simulink model "Final_Model_Building_2_AirflowAdded_BufferMode"  (R2022a)
settings: Solver=FixedStepAuto  StartTime=0.0  StopTime=24*3600  FixedStep=5  RelTol=1e-3
values from neighbouring files (symbols this model uses):
  Aux_Threshold = 52    [Setup_Code_EWASP_VC.m]
  buildingAge = 2005    [Setup_Code_EWASP_VC.m]
  ceilingHeight = 2.4    [Setup_Code_EWASP_VC.m]
  conductiveHconnectMatrix = [ ... (first row only)    [Setup_Code_EWASP_VC.m]
  cRoofGreen = 100000    [Setup_Code_EWASP_VC.m]
  Defrost_After_Time = 30    [Setup_Code_EWASP_VC.m]
  DHWDemandProfile = occFreegainHotwaterElecTestPassiveOcc3(:,3)    [Setup_Code_EWASP_VC.m]
  Elec_Max = Elec_Max*(30/24.2)    [Setup_Code_EWASP_VC.m]
  Elec_Mid = Elec_Mid*(30/24.2)    [Setup_Code_EWASP_VC.m]
  Elec_Min = Elec_Min*(30/24.2)    [Setup_Code_EWASP_VC.m]
  ElecDemandProfile = occFreegainHotwaterElecTestPassiveOcc3(:,4)    [Setup_Code_EWASP_VC.m]
  ElecFixed = [Elec_Max(6,2) Elec_Max(6,4) Elec_Max(6,6) Elec_Max(6,7) ... (first row only)    [Setup_Code_EWASP_VC.m]
  floorOrCeilingArea = floorOrCeilingArea*1.15    [Setup_Code_EWASP_VC.m]
  freegain = occFreegainHotwaterElecTestPassiveOcc3(:,2)-max(occupancy)*25    [Setup_Code_EWASP_VC.m]
  furnitureModelOn = 1    [Setup_Code_EWASP_VC.m]
  Heat_Max = Heat_Max*(30/24.2)    [Setup_Code_EWASP_VC.m]
  Heat_Mid = Heat_Mid*(30/24.2)    [Setup_Code_EWASP_VC.m]
  Heat_Min = Heat_Min*(30/24.2)    [Setup_Code_EWASP_VC.m]
  HeatFixed = [Heat_Max(6,2) Heat_Max(6,4) Heat_Max(6,6) Heat_Max(6,7) ... (first row only)    [Setup_Code_EWASP_VC.m]
  HeatingOnProfile = repmat(HeatingOnProfile,365,1)    [Setup_Code_EWASP_VC.m]
  HEX_ReturnLowerLimit = 52.5    [Setup_Code_EWASP_VC.m]
  HEX_ReturnUpperLimit = 55    [Setup_Code_EWASP_VC.m]
  LeakMultiplier = 1+(2*(rand()-0.5)/10)    [Setup_Code_EWASP_VC.m]
  maxOcc = max(occupancyProfile)    [Setup_Code_EWASP_VC.m]
  NESW_wallArea = max(NESW_Lengths*ceilingHeight-NESW_Windows,0)    [Setup_Code_EWASP_VC.m]
  NESW_Windows = [ ... (first row only)    [Setup_Code_EWASP_VC.m]
  numRooms = roomCount    [Setup_Code_EWASP_VC.m]
  occupancy = occupancyProfile    [Setup_Code_EWASP_VC.m]
  offsetDays = 0    [Setup_Code_EWASP_VC.m]
  overChargeSeries = repmat(overChargeSeries,365,1)    [Setup_Code_EWASP_VC.m]
  pumpChoice = pumpChoices(MinIndex,1)    [Setup_Code_EWASP_VC.m]
  pumpRamp = 180    [Setup_Code_EWASP_VC.m]
  RoofIrradiance = Flat_NS_EW_RoofIrradiance(:,1)    [Setup_Code_EWASP_VC.m]
  roofStartTemp = ones(11,1)*20    [Setup_Code_EWASP_VC.m]
  rooftype = 0    [Setup_Code_EWASP_VC.m]
  RoomDataMatrix = [zeros(1,12);ones(1,12)*wallDensity;zeros(1,12);ones(1,12)*wallU;ones(1,12)*windowU;ones(1,12)*floorU;ones(1,12)*ceilingU;zeros(1,12);windowArea, 0;floorOrCeilingArea;zeros(1,12);floorOrCeilingArea*ceilingHeight]    [Setup_Code_EWASP_VC.m]
  roomVol = roomVol*1.15    [Setup_Code_EWASP_VC.m]
  slabStartTemp = (GroundTempTimeSeries(offsetDays*1440+1,1)+thermostatSetting)/2    [Setup_Code_EWASP_VC.m]
  SlackRequest = zeros(1440,1)    [Setup_Code_EWASP_VC.m]
  SolarThermalExists = 0    [Setup_Code_EWASP_VC.m]
  SourceFixed = HeatFixed-ElecFixed    [Setup_Code_EWASP_VC.m]
  StateSeries = StateSeriesGenerator(22,7,1)    [Setup_Code_EWASP_VC.m]
  Tank_Lower_Temp = 49.5    [Setup_Code_EWASP_VC.m]
  Tank_Upper_Temp = 52    [Setup_Code_EWASP_VC.m]
  Tank_Volume_m3 = 0.15    [Setup_Code_EWASP_VC.m]
  TankHeatHour = randi([1 5])-1    [Setup_Code_EWASP_VC.m]
  upDown = [0;0;0;0;1;1;1;1;1;1;1]    [Setup_Code_EWASP_VC.m]
  wallStartTempExt = thermostatSetting*(0.266+0.00215*outdoorStartTemp+0.018*wallU+0.00113*outdoorStartTemp*wallU+0.0068*wallU^2)    [Setup_Code_EWASP_VC.m]
undefined symbols (not defined in the file or in its folder): a, ceilingU, condUDMatrix, convUDMatrix, deltaPEXPANDED_E, deltaPEXPANDED_E2, deltaPEXPANDED_N, deltaPEXPANDED_N2, deltaPEXPANDED_S, deltaPEXPANDED_S2, deltaPEXPANDED_W, deltaPEXPANDED_W2, DesiredDHWTemp, DesiredFlowTempVsInOutDeltaTemp, DiffuseHorizontal, DiscIntNeverNeededParam, DNI, dwnAndConcrete, ExtractRates, GroundTempTimeSeries, HCM, HCM2, HCM_closed, HCM_closed2, intermediateU, IsTop, massFlowMatrix, mechEfficiency, neighbourMatrix, numericalRoomUse, RadiatorMatrix, room2roomflowmatrix_E, room2roomflowmatrix_E2, room2roomflowmatrix_N, room2roomflowmatrix_N2, room2roomflowmatrix_S, room2roomflowmatrix_S2, room2roomflowmatrix_W, room2roomflowmatrix_W2, StateAirInEXPANDED_E, StateAirInEXPANDED_E2, StateAirInEXPANDED_N, StateAirInEXPANDED_N2, StateAirInEXPANDED_S, StateAirInEXPANDED_S2, StateAirInEXPANDED_W, StateAirInEXPANDED_W2, StateAirOutEXPANDED_E, StateAirOutEXPANDED_E2, StateAirOutEXPANDED_N, StateAirOutEXPANDED_N2, StateAirOutEXPANDED_S, StateAirOutEXPANDED_S2, StateAirOutEXPANDED_W, StateAirOutEXPANDED_W2, tankExists, TemperatureSeries, ThermostatBand, ThermostatSetting, Tin1 ... (+10)
libraries: simulink x6, dspsigops x4, dspmtrx3 x4, powerlib_meascontrol x3, carnot x3, dspstat3 x2
(part 3 of 29)

== system Final_Model_Building_2_AirflowAdded_BufferMode/Subsystem4 ==
  note: roof masses (45kg/m^2) and heat capacities calculated
      | using https://www.steelbeamcalculator.co.uk/standardloads
  In1 : Inport
  In2 : Inport  Port=2
  In3 : Inport  Port=3
  Ceil node tmperatures : DiscreteIntegrator  InitialConditionSource=external  InitialCondition=20  SampleTime=-1  ICPrevOutput=DiscIntNeverNeededParam  ICPrevScaledInput=DiscIntNeverNeededParam
  Display1 : Display
  Divide : Product  Inputs=*/
  Divide1 : Product  Inputs=*/
  Heat to ceilingNodes : Product  Inputs=4
  Heat to roofspace airnode : Sum  Inputs=+
  Heatloss roof to environment : Subsystem
  MATLAB Function1 : MATLAB Function  TreatAsAtomicUnit=on
  MATLAB Function2 : MATLAB Function  TreatAsAtomicUnit=on
  MATLAB Function3 : MATLAB Function  TreatAsAtomicUnit=on
  MATLAB Function4 : MATLAB Function  TreatAsAtomicUnit=on
  Product1 : Product  Inputs=3
  "Roof Temp " : DiscreteIntegrator  InitialConditionSource=external  InitialCondition=20  SampleTime=-1  ICPrevOutput=DiscIntNeverNeededParam  ICPrevScaledInput=DiscIntNeverNeededParam
  "RoofspaceTemp " : DiscreteIntegrator  InitialConditionSource=external  InitialCondition=20  SampleTime=-1  ICPrevOutput=DiscIntNeverNeededParam  ICPrevScaledInput=DiscIntNeverNeededParam
  Subtract : Sum  Inputs=+-
  Subtract1 : Sum
  Subtract2 : Sum  Inputs=+-
  Subtract3 : Sum  Inputs=+-
  Subtract4 : Sum  Inputs=2
  Subtract5 : Sum  Inputs=-+
  Total roofstructure heat capacity : Product
  Unary Minus : UnaryMinus
  air density per m3 : Constant  Value=1.225
  air heat capacity per kg : Constant  Value=1000
  ceiling heatchange due to loss to roofspace : UnaryMinus
  ceilnode heat capacities(predominantly plaster mass) : Constant  Value=10*1090*(IsTop(1:1:11)').*floorOrCeilingArea(1:1:11)'
  ceilnode heat capacities(predominantly plaster mass)1 : Constant  Value=10*1090*(IsTop(1,1:11)').*floorOrCeilingArea(1,1:11)'
  convective transfer to ceiling node : Constant  Value=2
  deltaTCeilingNodes : Product  Inputs=*/
  deltaTCeilingNodes1 : Product  Inputs=*/
  estimate of pitched roofspace air volume: 0.5 * floorArea of loft * height at peak : Constant  Value=0.5*sum(floorOrCeilingArea(1,1:11)'.*IsTop(1,1:11)')*(0.5*(sum(floorOrCeilingArea(1,1:11)'.*IsTop(1,1:11)')).^0.5)
  heat loss ceiing to roofspace : Product
  heat loss roofspace to roof : Product
  initial ceilnode temps : Constant  Value=20*ones(11,1)
  initial ceilnode temps1 : Constant  Value=10
  initial ceilnode temps2 : Constant  Value=10
  mass of roof per m^2*predictedroofarea : Constant  Value=45*sum(floorOrCeilingArea(1,1:11)'.*IsTop(1,1:11)')*1.414
  roofspace heatchange due to loss to roof : UnaryMinus
  room is on the top floor : Constant  Value=IsTop(1,1:11)'
  room is on the top floor1 : Constant  Value=floorOrCeilingArea(1,1:11)'
  slate heat capacity per kg1 : Constant  Value=760
  w/k loss from ceiling to roofspace : Constant  Value=(ceilingU*2)*(floorOrCeilingArea(1,1:11)').*(IsTop(1,1:11)')
  w/k loss from roofspace to roof : Constant  Value=(ceilingU*2)*sum(floorOrCeilingArea(1,1:11)'.*IsTop(1,1:11)')*1.414
  Out1 : Outport  VectorParamsAs1DForOutWhenUnconnected=off
  wires:
  In2/1 -> [windSpeed]
  In1/1 -> Subtract/1
  Subtract5/1 -> Divide1/1
  w/k loss from roofspace to roof/1 -> heat loss roofspace to roof/2
  Subtract/1 -> Heat to ceilingNodes/1
  Product1/1 -> Divide/2
  estimate of pitched roofspace air volume: 0.5 * floorArea of loft * height at peak/1 -> Product1/2
  air heat capacity per kg/1 -> Product1/3
  room is on the top floor/1 -> Heat to ceilingNodes/2
  heat loss roofspace to roof/1 -> roofspace heatchange due to loss to roof/1, Subtract5/2
  MATLAB Function3/1(y) -> Subtract1/2
  convective transfer to ceiling node/1 -> Heat to ceilingNodes/4
  air density per m3/1 -> Product1/1
  initial ceilnode temps1/1 -> "RoofspaceTemp "/2
  Heatloss roof to environment/1(Out1) -> Subtract5/1
  Heat to roofspace airnode/1 -> Display1/1, Subtract4/1
  Total roofstructure heat capacity/1 -> Divide1/2
  slate heat capacity per kg1/1 -> Total roofstructure heat capacity/1
  deltaTCeilingNodes1/1 -> MATLAB Function3/1(u)
  ceilnode heat capacities(predominantly plaster mass)1/1 -> deltaTCeilingNodes1/2
  MATLAB Function4/1(y) -> "Roof Temp "/1
  w/k loss from ceiling to roofspace/1 -> heat loss ceiing to roofspace/2
  deltaTCeilingNodes/1 -> MATLAB Function1/1(u)
  Subtract4/1 -> Divide/1
  Subtract3/1 -> heat loss roofspace to roof/1
  MATLAB Function2/1(y) -> "RoofspaceTemp "/1
  room is on the top floor1/1 -> Heat to ceilingNodes/3
  Ceil node tmperatures/1 -> Subtract2/1, Subtract/2
  mass of roof per m^2*predictedroofarea/1 -> Total roofstructure heat capacity/2
  ceilnode heat capacities(predominantly plaster mass)/1 -> deltaTCeilingNodes/2
  ceiling heatchange due to loss to roofspace/1 -> deltaTCeilingNodes1/1
  [windSpeed] -> Heatloss roof to environment/1(In1)
  initial ceilnode temps2/1 -> "Roof Temp "/2
  Heat to ceilingNodes/1 -> Unary Minus/1, deltaTCeilingNodes/1
  MATLAB Function1/1(y) -> Subtract1/1
  In3/1 -> [outdoorTemp]
  roofspace heatchange due to loss to roof/1 -> Subtract4/2
  Subtract2/1 -> heat loss ceiing to roofspace/1
  Divide1/1 -> MATLAB Function4/1(u)
  Divide/1 -> MATLAB Function2/1(u)
  "RoofspaceTemp "/1 -> Subtract3/1, Subtract2/2
  [outdoorTemp] -> Heatloss roof to environment/2(In2)
  Subtract1/1 -> Ceil node tmperatures/1
  initial ceilnode temps/1 -> Ceil node tmperatures/2
  heat loss ceiing to roofspace/1 -> ceiling heatchange due to loss to roofspace/1, Heat to roofspace airnode/1
  "Roof Temp "/1 -> Subtract3/2, Heatloss roof to environment/3(In3)
  Unary Minus/1 -> Out1/1

== system Final_Model_Building_2_AirflowAdded_BufferMode/Subsystem_Room1 ==
  DNI1 : Constant  Value=50
  Diffuse Irradiance1 : Constant  Value=50
  Ground : Ground
  Incidence Angle1 : Constant  Value=60
  Integrator : Integrator  InitialConditionSource=external  InitialCondition=Tin1
  Lounge/Dining : Subsystem
      mask Display:
      | port_label('input', 1, 'THB in')
      | port_label('input', 2, 'Mdot_Rad_Full_open')
      | port_label('input', 3, 'T In')
      | port_label('input', 4, 'T Out')
      | port_label('input', 5, 'T up (conv)')
      | port_label('input', 6, 'T Down (conv)')
      | port_label('input', 7, 'T Bel (cond)')
      | port_label('input', 8, 'T Abv (cond)')
      | port_label('input', 9, 'T N1')
      | port_label('input', 10, 'T N2')
      | port_label('input', 11, 'T N3')
      | port_label('input', 12, 'T N4')
      | port_label('input', 13, 'T N5')
      | port_label('input', 14, 'T Wall')
      | port_label('input', 15, 'Ang')
      | port_label('input', 16, 'Tilt')
      | port_label('input', 17, 'DNI')
      | port_label('input', 18, 'DiffI')
      | 
      | port_label('output', 1, 'THB Out')
      | port_label('output', 2, 'DeltaT Wall')
      | port_label('output', 3, 'DeltaT Room')
      | port_label('output', 5, 'Mdot_Actual')
  Panel TIlt1 : Constant  Value=90
  Subsystem11 : Subsystem
      mask Display:
      | disp('Vertical \n Conductive \n Signalling \n Block')
      | port_label('input', 1, 'Bel1')
      | port_label('input', 2, 'Bel2')
      | port_label('input', 3, 'Abv1')
      | port_label('input', 4, 'Abv2')
      | 
      | port_label('output', 1, 'T Bel')
      | port_label('output', 2, 'T Abv')
  Subsystem3 : Subsystem
      mask Display:
      | disp('Horizontal \n Neighbour \n Signalling \n Block')
      | port_label('input', 1, 'Nbr1')
      | port_label('input', 2, 'Nbr2')
      | port_label('input', 3, 'Nbr3')
      | port_label('input', 4, 'Nbr4')
      | port_label('input', 5, 'Nbr5')
      | port_label('output', 1, 'TN1')
      | port_label('output', 2, 'TN2')
      | port_label('output', 3, 'TN3')
      | port_label('output', 4, 'TN4')
      | port_label('output', 5, 'TN5')
  Terminator14 : Terminator
  Terminator2 : Terminator
  Tinitial1 : Constant  Value=21
  Twall11 : Constant  Value=neighbourMatrix(1,1)
  Twall12 : Constant  Value=neighbourMatrix(2,1)
  Twall13 : Constant  Value=neighbourMatrix(3,1)
  Twall14 : Constant  Value=neighbourMatrix(4,1)
  Twall15 : Constant  Value=neighbourMatrix(5,1)
  Twall33 : Constant  Value=condUDMatrix(1,1)
  Twall34 : Constant  Value=condUDMatrix(2,1)
  Twall35 : Constant  Value=condUDMatrix(3,1)
  Twall36 : Constant  Value=condUDMatrix(4,1)
  tag scope: DeltaT_1=global, Mdot_Actual_1=global, T_1=global, T_return_R1=global
  wires:
  [T_Out] -> Lounge/Dining/4(In3)
  Subsystem11/1(Out1) -> Lounge/Dining/7(In6)
  [T_1] -> Lounge/Dining/3(In2)
  Incidence Angle1/1 -> Lounge/Dining/15(In14)
  DNI1/1 -> Lounge/Dining/17(In16)
  Twall34/1 -> Subsystem11/2(In2)
  Subsystem3/5(Out5) -> Lounge/Dining/13(In12)
  Twall36/1 -> Subsystem11/4(In4)
  Twall33/1 -> Subsystem11/1(In1)
  Tinitial1/1 -> Integrator/2
  [DeltaT_1] -> Integrator/1
  [T_1] -> Lounge/Dining/5(In4), Lounge/Dining/6(In5)
  Twall11/1 -> Subsystem3/1(In1)
  Lounge/Dining/5(Out5) -> [Mdot_Actual_1]
  Subsystem3/1(Out1) -> Lounge/Dining/9(In8)
  Lounge/Dining/3(Out3) -> [DeltaT_1]
  Lounge/Dining/1(Out1) -> [T_return_R1]
  Lounge/Dining/4(Out4) -> Terminator2/1
  Diffuse Irradiance1/1 -> Lounge/Dining/18(In17)
  Lounge/Dining/2(Out2) -> Terminator14/1
  [THB_In] -> Lounge/Dining/1(In1)
  [MassFlow_Full_Open_1] -> Lounge/Dining/2(In18)
  Subsystem3/4(Out4) -> Lounge/Dining/12(In11)
  Twall13/1 -> Subsystem3/3(In3)
  Subsystem3/3(Out3) -> Lounge/Dining/11(In10)
  Twall15/1 -> Subsystem3/5(In5)
  Subsystem11/2(Out2) -> Lounge/Dining/8(In7)
  Ground/1 -> Lounge/Dining/14(In13)
  Twall14/1 -> Subsystem3/4(In4)
  Panel TIlt1/1 -> Lounge/Dining/16(In15)
  Integrator/1 -> [T_1]
  Twall12/1 -> Subsystem3/2(In2)
  Subsystem3/2(Out2) -> Lounge/Dining/10(In9)
  Twall35/1 -> Subsystem11/3(In3)

== system Final_Model_Building_2_AirflowAdded_BufferMode/Subsystem_Room10 ==
  DNI15 : Constant  Value=0
  Diffuse Irradiance10 : Constant  Value=0
  En suite : Subsystem
      mask Display:
      | port_label('input', 1, 'THB in')
      | port_label('input', 2, 'T In')
      | port_label('input', 3, 'T Out')
      | port_label('input', 4, 'T up (conv)')
      | port_label('input', 5, 'T Down (conv)')
      | port_label('input', 6, 'T Bel (cond)')
      | port_label('input', 7, 'T Abv (cond)')
      | port_label('input', 8, 'T N1')
      | port_label('input', 9, 'T N2')
      | port_label('input', 10, 'T N3')
      | port_label('input', 11, 'T N4')
      | port_label('input', 12, 'T N5')
      | port_label('input', 13, 'T Wall')
      | port_label('input', 14, 'Ang')
      | port_label('input', 15, 'Tilt')
      | port_label('input', 16, 'DNI')
      | port_label('input', 17, 'DiffI')
      | 
      | port_label('output', 1, 'THB Out')
      | port_label('output', 2, 'DeltaT Wall')
      | port_label('output', 3, 'DeltaT Room')
      | 
      | port_label('input', 18, 'm_dot_Fully_open')
      | port_label('output', 5, 'm_dot_Actual')
  Ground6 : Ground
  Incidence Angle10 : Constant  Value=60
  Integrator20 : Integrator  InitialConditionSource=external  InitialCondition=Tin1
  Panel TIlt10 : Constant  Value=90
  Scope34 : Scope
  Subsystem12 : Subsystem
      mask Display:
      | disp('Horizontal \n Neighbour \n Signalling \n Block')
      | port_label('input', 1, 'Nbr1')
      | port_label('input', 2, 'Nbr2')
      | port_label('input', 3, 'Nbr3')
      | port_label('input', 4, 'Nbr4')
      | port_label('input', 5, 'Nbr5')
      | port_label('output', 1, 'TN1')
      | port_label('output', 2, 'TN2')
      | port_label('output', 3, 'TN3')
      | port_label('output', 4, 'TN4')
      | port_label('output', 5, 'TN5')
  Subsystem23 : Subsystem
      mask Display:
      | disp('Vertical \n Convective \n Signalling \n Block')
      | port_label('input', 1, 'Nbr1')
      | port_label('input', 2, 'Nbr2')
      | 
      | port_label('output', 1, 'Tup')
      | port_label('output', 2, 'Tdwn')
  Subsystem28 : Subsystem
      mask Display:
      | disp('Vertical \n Conductive \n Signalling \n Block')
      | port_label('input', 1, 'Bel1')
      | port_label('input', 2, 'Bel2')
      | port_label('input', 3, 'Abv1')
      | port_label('input', 4, 'Abv2')
      | 
      | port_label('output', 1, 'T Bel')
      | port_label('output', 2, 'T Abv')
  Terminator7 : Terminator
  Tinitial14 : Constant  Value=20
  Twall100 : Constant  Value=condUDMatrix(1,10)
  Twall101 : Constant  Value=condUDMatrix(2,10)
  Twall102 : Constant  Value=condUDMatrix(3,10)
  Twall103 : Constant  Value=condUDMatrix(4,10)
  Twall51 : Constant  Value=neighbourMatrix(1,10)
  Twall52 : Constant  Value=neighbourMatrix(2,10)
  Twall53 : Constant  Value=neighbourMatrix(3,10)
  Twall54 : Constant  Value=neighbourMatrix(4,10)
  Twall55 : Constant  Value=neighbourMatrix(5,10)
  Twall82 : Constant  Value=convUDMatrix(1,10)
  Twall83 : Constant  Value=convUDMatrix(2,10)
  tag scope: DeltaT_10=global, Mdot_Actual_10=global, T_10=global, T_return_R10=global
  wires:
  Tinitial14/1 -> Integrator20/2
  [DeltaT_10] -> Integrator20/1
  Ground6/1 -> En suite/13(In13)
  Subsystem12/1(Out1) -> En suite/8(In8)
  [MassFlow_Full_Open_10] -> En suite/18(In18)
  DNI15/1 -> En suite/16(In16)
  Twall82/1 -> Subsystem23/1(In1)
  Subsystem12/4(Out4) -> En suite/11(In11)
  Panel TIlt10/1 -> En suite/15(In15)
  Subsystem28/2(Out2) -> En suite/7(In7)
  Twall55/1 -> Subsystem12/5(In5)
  [THB_In] -> En suite/1(In1)
  Diffuse Irradiance10/1 -> En suite/17(In17)
  En suite/3(Out3) -> [DeltaT_10]
  Twall83/1 -> Subsystem23/2(In2)
  En suite/2(Out2) -> Terminator7/1
  En suite/5(Out5) -> [Mdot_Actual_10]
  En suite/1(Out1) -> [T_return_R10]
  Incidence Angle10/1 -> En suite/14(In14)
  Twall102/1 -> Subsystem28/3(In3)
  [T_10] -> En suite/2(In2)
  Twall53/1 -> Subsystem12/3(In3)
  Integrator20/1 -> [T_10]
  Subsystem12/2(Out2) -> En suite/9(In9)
  Subsystem23/2(Out2) -> En suite/5(In5)
  Subsystem12/3(Out3) -> En suite/10(In10)
  En suite/4(Out4) -> Scope34/1
  Subsystem23/1(Out1) -> En suite/4(In4)
  Twall54/1 -> Subsystem12/4(In4)
  Twall100/1 -> Subsystem28/1(In1)
  Subsystem12/5(Out5) -> En suite/12(In12)
  Twall52/1 -> Subsystem12/2(In2)
  [T_Out] -> En suite/3(In3)
  Twall103/1 -> Subsystem28/4(In4)
  Twall51/1 -> Subsystem12/1(In1)
  Subsystem28/1(Out1) -> En suite/6(In6)
  Twall101/1 -> Subsystem28/2(In2)

== system Final_Model_Building_2_AirflowAdded_BufferMode/Subsystem_Room11 ==
  Bathroom : Subsystem
      mask Display:
      | port_label('input', 1, 'THB in')
      | port_label('input', 2, 'T In')
      | port_label('input', 3, 'T Out')
      | port_label('input', 4, 'T up (conv)')
      | port_label('input', 5, 'T Down (conv)')
      | port_label('input', 6, 'T Bel (cond)')
      | port_label('input', 7, 'T Abv (cond)')
      | port_label('input', 8, 'T N1')
      | port_label('input', 9, 'T N2')
      | port_label('input', 10, 'T N3')
      | port_label('input', 11, 'T N4')
      | port_label('input', 12, 'T N5')
      | port_label('input', 13, 'T Wall')
      | port_label('input', 14, 'Ang')
      | port_label('input', 15, 'Tilt')
      | port_label('input', 16, 'DNI')
      | port_label('input', 17, 'DiffI')
      | 
      | port_label('output', 1, 'THB Out')
      | port_label('output', 2, 'DeltaT Wall')
      | port_label('output', 3, 'DeltaT Room')
      | 
      | port_label('input', 18, 'm_dot_Fully_open')
      | port_label('output', 5, 'm_dot_Actual')
  DNI9 : Constant  Value=0
  Diffuse Irradiance11 : Constant  Value=0
  Ground5 : Ground
  Incidence Angle11 : Constant  Value=60
  Integrator24 : Integrator  InitialConditionSource=external  InitialCondition=Tin1
  Panel TIlt11 : Constant  Value=90
  Scope33 : Scope
  Subsystem13 : Subsystem
      mask Display:
      | disp('Horizontal \n Neighbour \n Signalling \n Block')
      | port_label('input', 1, 'Nbr1')
      | port_label('input', 2, 'Nbr2')
      | port_label('input', 3, 'Nbr3')
      | port_label('input', 4, 'Nbr4')
      | port_label('input', 5, 'Nbr5')
      | port_label('output', 1, 'TN1')
      | port_label('output', 2, 'TN2')
      | port_label('output', 3, 'TN3')
      | port_label('output', 4, 'TN4')
      | port_label('output', 5, 'TN5')
  Subsystem24 : Subsystem
      mask Display:
      | disp('Vertical \n Convective \n Signalling \n Block')
      | port_label('input', 1, 'Nbr1')
      | port_label('input', 2, 'Nbr2')
      | 
      | port_label('output', 1, 'Tup')
      | port_label('output', 2, 'Tdwn')
  Subsystem29 : Subsystem
      mask Display:
      | disp('Vertical \n Conductive \n Signalling \n Block')
      | port_label('input', 1, 'Bel1')
      | port_label('input', 2, 'Bel2')
      | port_label('input', 3, 'Abv1')
      | port_label('input', 4, 'Abv2')
      | 
      | port_label('output', 1, 'T Bel')
      | port_label('output', 2, 'T Abv')
  Terminator8 : Terminator
  Tinitial15 : Constant  Value=20
  Twall123 : Constant  Value=condUDMatrix(1,11)
  Twall133 : Constant  Value=condUDMatrix(2,11)
  Twall134 : Constant  Value=condUDMatrix(3,11)
  Twall135 : Constant  Value=condUDMatrix(4,11)
  Twall56 : Constant  Value=neighbourMatrix(1,11)
  Twall57 : Constant  Value=neighbourMatrix(2,11)
  Twall58 : Constant  Value=neighbourMatrix(3,11)
  Twall59 : Constant  Value=neighbourMatrix(4,11)
  Twall60 : Constant  Value=neighbourMatrix(5,11)
  Twall84 : Constant  Value=convUDMatrix(1,11)
  Twall85 : Constant  Value=convUDMatrix(2,11)
  tag scope: DeltaT_11=global, Mdot_Actual_11=global, T_11=global, T_return_R11=global
  wires:
  Bathroom/1(Out1) -> [T_return_R11]
  [DeltaT_11] -> Integrator24/1
  [MassFlow_Full_Open_11] -> Bathroom/18(In18)
  Diffuse Irradiance11/1 -> Bathroom/17(In17)
  Subsystem13/1(Out1) -> Bathroom/8(In8)
  Subsystem13/3(Out3) -> Bathroom/10(In10)
  Subsystem13/2(Out2) -> Bathroom/9(In9)
  Subsystem24/2(Out2) -> Bathroom/5(In5)
  Bathroom/4(Out4) -> Scope33/1
  Subsystem13/4(Out4) -> Bathroom/11(In11)
  [T_11] -> Bathroom/2(In2)
  Twall57/1 -> Subsystem13/2(In2)
  Bathroom/3(Out3) -> [DeltaT_11]
  DNI9/1 -> Bathroom/16(In16)
  Twall58/1 -> Subsystem13/3(In3)
  Twall135/1 -> Subsystem29/4(In4)
  Twall84/1 -> Subsystem24/1(In1)
  Twall59/1 -> Subsystem13/4(In4)
  Tinitial15/1 -> Integrator24/2
  Twall123/1 -> Subsystem29/1(In1)
  Panel TIlt11/1 -> Bathroom/15(In15)
  Twall60/1 -> Subsystem13/5(In5)
  Subsystem24/1(Out1) -> Bathroom/4(In4)
  Twall85/1 -> Subsystem24/2(In2)
  Integrator24/1 -> [T_11]
  [T_Out] -> Bathroom/3(In3)
  Subsystem29/2(Out2) -> Bathroom/7(In7)
  Twall56/1 -> Subsystem13/1(In1)
  Bathroom/2(Out2) -> Terminator8/1
  [THB_In] -> Bathroom/1(In1)
  Bathroom/5(Out5) -> [Mdot_Actual_11]
  Twall134/1 -> Subsystem29/3(In3)
  Subsystem13/5(Out5) -> Bathroom/12(In12)
  Incidence Angle11/1 -> Bathroom/14(In14)
  Twall133/1 -> Subsystem29/2(In2)
  Subsystem29/1(Out1) -> Bathroom/6(In6)
  Ground5/1 -> Bathroom/13(In13)

== system Final_Model_Building_2_AirflowAdded_BufferMode/Subsystem_Room2 ==
  DNI2 : Constant  Value=0
  Diffuse Irradiance2 : Constant  Value=0
  Ground1 : Ground
  Incidence Angle2 : Constant  Value=60
  Integrator1 : Integrator  InitialConditionSource=external  InitialCondition=Tin1
  Kitchen : Subsystem
      mask Display:
      | port_label('input', 1, 'THB in')
      | port_label('input', 2, 'T In')
      | port_label('input', 3, 'T Out')
      | port_label('input', 4, 'T up (conv)')
      | port_label('input', 5, 'T Down (conv)')
      | port_label('input', 6, 'T Bel (cond)')
      | port_label('input', 7, 'T Abv (cond)')
      | port_label('input', 8, 'T N1')
      | port_label('input', 9, 'T N2')
      | port_label('input', 10, 'T N3')
      | port_label('input', 11, 'T N4')
      | port_label('input', 12, 'T N5')
      | port_label('input', 13, 'T Wall')
      | port_label('input', 14, 'Ang')
      | port_label('input', 15, 'Tilt')
      | port_label('input', 16, 'DNI')
      | port_label('input', 17, 'DiffI')
      | 
      | port_label('output', 1, 'THB Out')
      | 
      | port_label('output', 2, 'DeltaT Room')
      | 
      | port_label('input', 18, 'm_dot_Fully_open')
      | port_label('output', 3, 'm_dot_Actual')
  Panel TIlt2 : Constant  Value=90
  Subsystem10 : Subsystem
      mask Display:
      | disp('Vertical \n Conductive \n Signalling \n Block')
      | port_label('input', 1, 'Bel1')
      | port_label('input', 2, 'Bel2')
      | port_label('input', 3, 'Abv1')
      | port_label('input', 4, 'Abv2')
      | 
      | port_label('output', 1, 'T Bel')
      | port_label('output', 2, 'T Abv')
  Subsystem4 : Subsystem
      mask Display:
      | disp('Horizontal \n Neighbour \n Signalling \n Block')
      | port_label('input', 1, 'Nbr1')
      | port_label('input', 2, 'Nbr2')
      | port_label('input', 3, 'Nbr3')
      | port_label('input', 4, 'Nbr4')
      | port_label('input', 5, 'Nbr5')
      | port_label('output', 1, 'TN1')
      | port_label('output', 2, 'TN2')
      | port_label('output', 3, 'TN3')
      | port_label('output', 4, 'TN4')
      | port_label('output', 5, 'TN5')
  Terminator : Terminator
  Tinitial2 : Constant  Value=20
  Twall10 : Constant  Value=condUDMatrix(2,2)
  Twall128 : Constant  Value=neighbourMatrix(1,2)
  Twall129 : Constant  Value=neighbourMatrix(2,2)
  Twall130 : Constant  Value=neighbourMatrix(3,2)
  Twall131 : Constant  Value=neighbourMatrix(4,2)
  Twall132 : Constant  Value=neighbourMatrix(5,2)
  Twall31 : Constant  Value=condUDMatrix(3,3)
  Twall32 : Constant  Value=condUDMatrix(4,4)
  Twall9 : Constant  Value=condUDMatrix(1,2)
  tag scope: DeltaT_2=global, Mdot_Actual_2=global, T_2=global, T_return_R2=global
  wires:
  Subsystem10/2(Out2) -> Kitchen/7(In7)
  Twall9/1 -> Subsystem10/1(In1)
  Diffuse Irradiance2/1 -> Kitchen/17(In17)
  Twall10/1 -> Subsystem10/2(In2)
  Ground1/1 -> Kitchen/13(In13)
  [T_2] -> Kitchen/2(In2)
  [T_2] -> Kitchen/4(In4), Kitchen/5(In5)
  Subsystem4/3(Out3) -> Kitchen/10(In10)
  Subsystem10/1(Out1) -> Kitchen/6(In6)
  Twall32/1 -> Subsystem10/4(In4)
  [T_Out] -> Kitchen/3(In3)
  Incidence Angle2/1 -> Kitchen/14(In14)
  Twall31/1 -> Subsystem10/3(In3)
  Subsystem4/1(Out1) -> Kitchen/8(In8)
  Tinitial2/1 -> Integrator1/2
  Twall132/1 -> Subsystem4/5(In5)
  [DeltaT_2] -> Integrator1/1
  Twall130/1 -> Subsystem4/3(In3)
  Subsystem4/5(Out5) -> Kitchen/12(In12)
  Kitchen/2(Out3) -> [DeltaT_2]
  Kitchen/3(Out4) -> [Mdot_Actual_2]
  Kitchen/1(Out1) -> [T_return_R2]
  [MassFlow_Full_Open_2] -> Kitchen/18(In18)
  DNI2/1 -> Kitchen/16(In16)
  Subsystem4/2(Out2) -> Kitchen/9(In9)
  [THB_In] -> Kitchen/1(In1)
  Twall128/1 -> Subsystem4/1(In1)
  Twall131/1 -> Subsystem4/4(In4)
  Panel TIlt2/1 -> Kitchen/15(In15)
  Twall129/1 -> Subsystem4/2(In2)
  Integrator1/1 -> [T_2]
  Kitchen/4(Out2) -> Terminator/1
  Subsystem4/4(Out4) -> Kitchen/11(In11)

== system Final_Model_Building_2_AirflowAdded_BufferMode/Subsystem_Room3 ==
  DNI3 : Constant  Value=0
  Diffuse Irradiance3 : Constant  Value=50
  Ground2 : Ground
  Incidence Angle3 : Constant  Value=60
  Integrator5 : Integrator  InitialConditionSource=external  InitialCondition=Tin1
  Panel TIlt3 : Constant  Value=90
  Subsystem5 : Subsystem
      mask Display:
      | disp('Horizontal \n Neighbour \n Signalling \n Block')
      | port_label('input', 1, 'Nbr1')
      | port_label('input', 2, 'Nbr2')
      | port_label('input', 3, 'Nbr3')
      | port_label('input', 4, 'Nbr4')
      | port_label('input', 5, 'Nbr5')
      | port_label('output', 1, 'TN1')
      | port_label('output', 2, 'TN2')
      | port_label('output', 3, 'TN3')
      | port_label('output', 4, 'TN4')
      | port_label('output', 5, 'TN5')
  Subsystem9 : Subsystem
      mask Display:
      | disp('Vertical \n Conductive \n Signalling \n Block')
      | port_label('input', 1, 'Bel1')
      | port_label('input', 2, 'Bel2')
      | port_label('input', 3, 'Abv1')
      | port_label('input', 4, 'Abv2')
      | 
      | port_label('output', 1, 'T Bel')
      | port_label('output', 2, 'T Abv')
  Terminator11 : Terminator
  Tinitial3 : Constant  Value=20
  Twall16 : Constant  Value=neighbourMatrix(1,3)
  Twall17 : Constant  Value=neighbourMatrix(2,3)
  Twall18 : Constant  Value=neighbourMatrix(3,3)
  Twall19 : Constant  Value=neighbourMatrix(4,3)
  Twall20 : Constant  Value=neighbourMatrix(5,3)
  Twall5 : Constant  Value=condUDMatrix(1,3)
  Twall6 : Constant  Value=condUDMatrix(2,3)
  Twall7 : Constant  Value=condUDMatrix(3,3)
  Twall8 : Constant  Value=condUDMatrix(4,3)
  Utility : Subsystem
      mask Display:
      | port_label('input', 1, 'THB in')
      | port_label('input', 2, 'T In')
      | port_label('input', 3, 'T Out')
      | port_label('input', 4, 'T up (conv)')
      | port_label('input', 5, 'T Down (conv)')
      | port_label('input', 6, 'T Bel (cond)')
      | port_label('input', 7, 'T Abv (cond)')
      | port_label('input', 8, 'T N1')
      | port_label('input', 9, 'T N2')
      | port_label('input', 10, 'T N3')
      | port_label('input', 11, 'T N4')
      | port_label('input', 12, 'T N5')
      | port_label('input', 13, 'T Wall')
      | port_label('input', 14, 'Ang')
      | port_label('input', 15, 'Tilt')
      | port_label('input', 16, 'DNI')
      | port_label('input', 17, 'DiffI')
      | 
      | port_label('output', 1, 'THB Out')
      | port_label('output', 2, 'DeltaT Wall')
      | port_label('output', 3, 'DeltaT Room')
      | 
      | port_label('input', 18, 'm_dot_Fully_open')
      | port_label('output', 4, 'm_dot_Actual')
  tag scope: DeltaT_3=global, Mdot_Actual_3=global, T_3=global, T_return_R3=global
  wires:
  Ground2/1 -> Utility/13(In13)
  Subsystem5/3(Out3) -> Utility/10(In10)
  Twall5/1 -> Subsystem9/1(In1)
  Twall8/1 -> Subsystem9/4(In4)
  Twall6/1 -> Subsystem9/2(In2)
  Utility/2(Out2) -> Terminator11/1
  Twall7/1 -> Subsystem9/3(In3)
  [T_3] -> Utility/2(In2)
  Subsystem9/1(Out1) -> Utility/6(In6)
  Subsystem9/2(Out2) -> Utility/7(In7)
  Diffuse Irradiance3/1 -> Utility/17(In17)
  Integrator5/1 -> [T_3]
  Twall18/1 -> Subsystem5/3(In3)
  Incidence Angle3/1 -> Utility/14(In14)
  DNI3/1 -> Utility/16(In16)
  Panel TIlt3/1 -> Utility/15(In15)
  [THB_In] -> Utility/1(In1)
  Tinitial3/1 -> Integrator5/2
  Twall20/1 -> Subsystem5/5(In5)
  [T_Out] -> Utility/3(In3)
  [T_3] -> Utility/5(In5), Utility/4(In4)
  [MassFlow_Full_Open_3] -> Utility/18(In18)
  Utility/4(Out4) -> [Mdot_Actual_3]
  Utility/1(Out1) -> [T_return_R3]
  Twall16/1 -> Subsystem5/1(In1)
  Subsystem5/4(Out4) -> Utility/11(In11)
  Twall17/1 -> Subsystem5/2(In2)
  Subsystem5/2(Out2) -> Utility/9(In9)
  Utility/3(Out3) -> [DeltaT_3]
  Subsystem5/5(Out5) -> Utility/12(In12)
  [DeltaT_3] -> Integrator5/1
  Subsystem5/1(Out1) -> Utility/8(In8)
  Twall19/1 -> Subsystem5/4(In4)

== system Final_Model_Building_2_AirflowAdded_BufferMode/Subsystem_Room4 ==
  DNI11 : Constant  Value=0
  Diffuse Irradiance8 : Constant  Value=50
  Ground3 : Ground
  Hall : Subsystem
      mask Display:
      | port_label('input', 1, 'THB in')
      | port_label('input', 2, 'T In')
      | port_label('input', 3, 'T Out')
      | port_label('input', 4, 'T up (conv)')
      | port_label('input', 5, 'T Down (conv)')
      | port_label('input', 6, 'T Bel (cond)')
      | port_label('input', 7, 'T Abv (cond)')
      | port_label('input', 8, 'T N1')
      | port_label('input', 9, 'T N2')
      | port_label('input', 10, 'T N3')
      | port_label('input', 11, 'T N4')
      | port_label('input', 12, 'T N5')
      | port_label('input', 13, 'T Wall')
      | port_label('input', 14, 'Ang')
      | port_label('input', 15, 'Tilt')
      | port_label('input', 16, 'DNI')
      | port_label('input', 17, 'DiffI')
      | 
      | port_label('output', 1, 'THB Out')
      | port_label('output', 2, 'DeltaT Wall')
      | port_label('output', 3, 'DeltaT Room')
      | 
      | 
      | port_label('input', 18, 'm_dot_Fully_open')
      | port_label('output', 4, 'm_dot_Actual')
  Incidence Angle8 : Constant  Value=60
  Integrator21 : Integrator  InitialConditionSource=external  InitialCondition=Tin1
  Panel TIlt8 : Constant  Value=90
  Subsystem6 : Subsystem
      mask Display:
      | disp('Horizontal \n Neighbour \n Signalling \n Block')
      | port_label('input', 1, 'Nbr1')
      | port_label('input', 2, 'Nbr2')
      | port_label('input', 3, 'Nbr3')
      | port_label('input', 4, 'Nbr4')
      | port_label('input', 5, 'Nbr5')
      | port_label('output', 1, 'TN1')
      | port_label('output', 2, 'TN2')
      | port_label('output', 3, 'TN3')
      | port_label('output', 4, 'TN4')
      | port_label('output', 5, 'TN5')
  Subsystem8 : Subsystem
      mask Display:
      | disp('Vertical \n Conductive \n Signalling \n Block')
      | port_label('input', 1, 'Bel1')
      | port_label('input', 2, 'Bel2')
      | port_label('input', 3, 'Abv1')
      | port_label('input', 4, 'Abv2')
      | 
      | port_label('output', 1, 'T Bel')
      | port_label('output', 2, 'T Abv')
  Terminator10 : Terminator
  Tinitial11 : Constant  Value=20
  Twall1 : Constant  Value=condUDMatrix(1,4)
  Twall2 : Constant  Value=condUDMatrix(2,4)
  Twall21 : Constant  Value=neighbourMatrix(1,4)
  Twall22 : Constant  Value=neighbourMatrix(2,4)
  Twall23 : Constant  Value=neighbourMatrix(3,4)
  Twall24 : Constant  Value=neighbourMatrix(4,4)
  Twall25 : Constant  Value=neighbourMatrix(5,4)
  Twall3 : Constant  Value=condUDMatrix(3,4)
  Twall4 : Constant  Value=condUDMatrix(4,4)
  tag scope: DeltaT_4=global, Mdot_Actual_4=global, T_4=global, T_return_R4=global
  wires:
  Subsystem8/2(Out2) -> Hall/7(In7)
  Integrator21/1 -> [T_4]
  Subsystem6/1(Out1) -> Hall/8(In8)
  Ground3/1 -> Hall/13(In13)
  [DeltaT_4] -> Integrator21/1
  Incidence Angle8/1 -> Hall/14(In14)
  Subsystem8/1(Out1) -> Hall/6(In6)
  Panel TIlt8/1 -> Hall/15(In15)
  [THB_In] -> Hall/1(In1)
  Twall21/1 -> Subsystem6/1(In1)
  DNI11/1 -> Hall/16(In16)
  Diffuse Irradiance8/1 -> Hall/17(In17)
  Hall/4(Out4) -> [Mdot_Actual_4]
  Hall/3(Out3) -> [DeltaT_4]
  Twall25/1 -> Subsystem6/5(In5)
  [MassFlow_Full_Open_4] -> Hall/18(In18)
  Twall23/1 -> Subsystem6/3(In3)
  Subsystem6/5(Out5) -> Hall/12(In12)
  Twall4/1 -> Subsystem8/4(In4)
  Twall2/1 -> Subsystem8/2(In2)
  [T_4] -> Hall/5(In5)
  Hall/2(Out2) -> Terminator10/1
  [T_4] -> Hall/2(In2)
  Subsystem6/4(Out4) -> Hall/11(In11)
  Subsystem6/3(Out3) -> Hall/10(In10)
  Twall24/1 -> Subsystem6/4(In4)
  Twall22/1 -> Subsystem6/2(In2)
  Hall/1(Out1) -> [T_return_R4]
  Subsystem6/2(Out2) -> Hall/9(In9)
  Tinitial11/1 -> Integrator21/2
  [T_5] -> Hall/4(In4)
  Twall1/1 -> Subsystem8/1(In1)
  [T_Out] -> Hall/3(In3)
  Twall3/1 -> Subsystem8/3(In3)

== system Final_Model_Building_2_AirflowAdded_BufferMode/Subsystem_Room5 ==
  DNI4 : Constant  Value=0
  Diffuse Irradiance4 : Constant  Value=0
  Ground4 : Ground
  Incidence Angle4 : Constant  Value=60
  Integrator6 : Integrator  InitialConditionSource=external  InitialCondition=Tin1
  Landing : Subsystem
      mask Display:
      | port_label('input', 1, 'THB in')
      | port_label('input', 2, 'T In')
      | port_label('input', 3, 'T Out')
      | port_label('input', 4, 'T up (conv)')
      | port_label('input', 5, 'T Down (conv)')
      | port_label('input', 6, 'T Bel (cond)')
      | port_label('input', 7, 'T Abv (cond)')
      | port_label('input', 8, 'T N1')
      | port_label('input', 9, 'T N2')
      | port_label('input', 10, 'T N3')
      | port_label('input', 11, 'T N4')
      | port_label('input', 12, 'T N5')
      | port_label('input', 13, 'T Wall')
      | port_label('input', 14, 'Ang')
      | port_label('input', 15, 'Tilt')
      | port_label('input', 16, 'DNI')
      | port_label('input', 17, 'DiffI')
      | 
      | port_label('output', 1, 'THB Out')
      | port_label('output', 2, 'DeltaT Wall')
      | port_label('output', 3, 'DeltaT Room')
      | 
      | port_label('input', 18, 'm_dot_Fully_open')
      | port_label('output', 5, 'm_dot_Actual')
  Panel TIlt4 : Constant  Value=90
  Subsystem18 : Subsystem
      mask Display:
      | disp('Vertical \n Convective \n Signalling \n Block')
      | port_label('input', 1, 'Nbr1')
      | port_label('input', 2, 'Nbr2')
      | 
      | port_label('output', 1, 'Tup')
      | port_label('output', 2, 'Tdwn')
  Subsystem35 : Subsystem
      mask Display:
      | disp('Vertical \n Conductive \n Signalling \n Block')
      | port_label('input', 1, 'Bel1')
      | port_label('input', 2, 'Bel2')
      | port_label('input', 3, 'Abv1')
      | port_label('input', 4, 'Abv2')
      | 
      | port_label('output', 1, 'T Bel')
      | port_label('output', 2, 'T Abv')
  Subsystem7 : Subsystem
      mask Display:
      | disp('Horizontal \n Neighbour \n Signalling \n Block')
      | port_label('input', 1, 'Nbr1')
      | port_label('input', 2, 'Nbr2')
      | port_label('input', 3, 'Nbr3')
      | port_label('input', 4, 'Nbr4')
      | port_label('input', 5, 'Nbr5')
      | port_label('output', 1, 'TN1')
      | port_label('output', 2, 'TN2')
      | port_label('output', 3, 'TN3')
      | port_label('output', 4, 'TN4')
      | port_label('output', 5, 'TN5')
  Terminator12 : Terminator
  Terminator9 : Terminator
  Tinitial4 : Constant  Value=20
  Twall104 : Constant  Value=convUDMatrix(1,5)
  Twall105 : Constant  Value=convUDMatrix(2,5)
  Twall119 : Constant  Value=condUDMatrix(1,5)
  Twall120 : Constant  Value=condUDMatrix(2,5)
  Twall121 : Constant  Value=condUDMatrix(3,5)
  Twall122 : Constant  Value=condUDMatrix(4,5)
  Twall26 : Constant  Value=neighbourMatrix(1,5)
  Twall27 : Constant  Value=neighbourMatrix(2,5)
  Twall28 : Constant  Value=neighbourMatrix(3,5)
  Twall29 : Constant  Value=neighbourMatrix(4,5)
  Twall30 : Constant  Value=neighbourMatrix(5,5)
  tag scope: DeltaT_5=global, Mdot_Actual_5=global, T_5=global, T_return_R5=global
  wires:
  DNI4/1 -> Landing/16(In16)
  Twall120/1 -> Subsystem35/2(In2)
  Tinitial4/1 -> Integrator6/2
  [DeltaT_5] -> Integrator6/1
  Landing/3(Out3) -> [DeltaT_5]
  Subsystem7/5(Out5) -> Landing/12(In12)
  Integrator6/1 -> [T_5]
  Subsystem7/1(Out1) -> Landing/8(In8)
  Twall119/1 -> Subsystem35/1(In1)
  Diffuse Irradiance4/1 -> Landing/17(In17)
  Panel TIlt4/1 -> Landing/15(In15)
  [THB_In] -> Landing/1(In1)
  [T_Out] -> Landing/3(In3)
  Landing/5(Out5) -> [Mdot_Actual_5]
  Incidence Angle4/1 -> Landing/14(In14)
  Subsystem35/1(Out1) -> Landing/6(In6)
  Twall26/1 -> Subsystem7/1(In1)
  [T_5] -> Landing/2(In2)
  Ground4/1 -> Landing/13(In13)
  Subsystem7/3(Out3) -> Landing/10(In10)
  [MassFlow_Full_Open_5] -> Landing/18(In18)
  Twall27/1 -> Subsystem7/2(In2)
  Twall121/1 -> Subsystem35/3(In3)
  Subsystem18/2(Out2) -> Landing/5(In5)
  Subsystem18/1(Out1) -> Landing/4(In4)
  Twall122/1 -> Subsystem35/4(In4)
  Landing/4(Out4) -> Terminator12/1
  Landing/2(Out2) -> Terminator9/1
  Twall105/1 -> Subsystem18/2(In2)
  Subsystem7/4(Out4) -> Landing/11(In11)
  Subsystem35/2(Out2) -> Landing/7(In7)
  Landing/1(Out1) -> [T_return_R5]
  Twall30/1 -> Subsystem7/5(In5)
  Twall28/1 -> Subsystem7/3(In3)
  Twall104/1 -> Subsystem18/1(In1)
  Twall29/1 -> Subsystem7/4(In4)
  Subsystem7/2(Out2) -> Landing/9(In9)

== system Final_Model_Building_2_AirflowAdded_BufferMode/Subsystem_Room6 ==
  Bedroom1 : Subsystem
      mask Display:
      | port_label('input', 1, 'THB in')
      | port_label('input', 2, 'T In')
      | port_label('input', 3, 'T Out')
      | port_label('input', 4, 'T up (conv)')
      | port_label('input', 5, 'T Down (conv)')
      | port_label('input', 6, 'T Bel (cond)')
      | port_label('input', 7, 'T Abv (cond)')
      | port_label('input', 8, 'T N1')
      | port_label('input', 9, 'T N2')
      | port_label('input', 10, 'T N3')
      | port_label('input', 11, 'T N4')
      | port_label('input', 12, 'T N5')
      | port_label('input', 13, 'T Wall')
      | port_label('input', 14, 'Ang')
      | port_label('input', 15, 'Tilt')
      | port_label('input', 16, 'DNI')
      | port_label('input', 17, 'DiffI')
      | 
      | port_label('output', 1, 'THB Out')
      | port_label('output', 2, 'DeltaT Wall')
      | port_label('output', 3, 'DeltaT Room')
      | 
      | port_label('input', 18, 'm_dot_Fully_open')
      | port_label('output', 5, 'm_dot_Actual')
  DNI5 : Constant  Value=0
  Diffuse Irradiance5 : Constant  Value=0
  Ground10 : Ground
  Incidence Angle5 : Constant  Value=60
  Integrator7 : Integrator  InitialConditionSource=external  InitialCondition=Tin1
  Panel TIlt5 : Constant  Value=90
  Scope38 : Scope
  Subsystem19 : Subsystem
      mask Display:
      | disp('Vertical \n Convective \n Signalling \n Block')
      | port_label('input', 1, 'Nbr1')
      | port_label('input', 2, 'Nbr2')
      | 
      | port_label('output', 1, 'Tup')
      | port_label('output', 2, 'Tdwn')
  Subsystem30 : Subsystem
      mask Display:
      | disp('Vertical \n Conductive \n Signalling \n Block')
      | port_label('input', 1, 'Bel1')
      | port_label('input', 2, 'Bel2')
      | port_label('input', 3, 'Abv1')
      | port_label('input', 4, 'Abv2')
      | 
      | port_label('output', 1, 'T Bel')
      | port_label('output', 2, 'T Abv')
  Subsystem8 : Subsystem
      mask Display:
      | disp('Horizontal \n Neighbour \n Signalling \n Block')
      | port_label('input', 1, 'Nbr1')
      | port_label('input', 2, 'Nbr2')
      | port_label('input', 3, 'Nbr3')
      | port_label('input', 4, 'Nbr4')
      | port_label('input', 5, 'Nbr5')
      | port_label('output', 1, 'TN1')
      | port_label('output', 2, 'TN2')
      | port_label('output', 3, 'TN3')
      | port_label('output', 4, 'TN4')
      | port_label('output', 5, 'TN5')
  Terminator4 : Terminator
  Tinitial5 : Constant  Value=20
  Twall108 : Constant  Value=condUDMatrix(1,6)
  Twall109 : Constant  Value=condUDMatrix(2,6)
  Twall110 : Constant  Value=condUDMatrix(3,6)
  Twall111 : Constant  Value=condUDMatrix(4,6)
  Twall31 : Constant  Value=neighbourMatrix(1,6)
  Twall32 : Constant  Value=neighbourMatrix(2,6)
  Twall33 : Constant  Value=neighbourMatrix(3,6)
  Twall34 : Constant  Value=neighbourMatrix(4,6)
  Twall35 : Constant  Value=neighbourMatrix(5,6)
  Twall74 : Constant  Value=convUDMatrix(1,6)
  Twall75 : Constant  Value=convUDMatrix(2,6)
  tag scope: DeltaT_6=global, Mdot_Actual_6=global, T_6=global, T_return_R6=global
  wires:
  Twall75/1 -> Subsystem19/2(In2)
  Subsystem8/1(Out1) -> Bedroom1/8(In8)
  DNI5/1 -> Bedroom1/16(In16)
  Subsystem19/2(Out2) -> Bedroom1/5(In5)
  [THB_In] -> Bedroom1/1(In1)
  Integrator7/1 -> [T_6]
  [T_6] -> Bedroom1/2(In2)
  Twall31/1 -> Subsystem8/1(In1)
  [DeltaT_6] -> Integrator7/1
  Subsystem19/1(Out1) -> Bedroom1/4(In4)
  Twall34/1 -> Subsystem8/4(In4)
  Incidence Angle5/1 -> Bedroom1/14(In14)
  Twall108/1 -> Subsystem30/1(In1)
  Ground10/1 -> Bedroom1/13(In13)
  [T_Out] -> Bedroom1/3(In3)
  Panel TIlt5/1 -> Bedroom1/15(In15)
  Bedroom1/3(Out3) -> [DeltaT_6]
  Bedroom1/4(Out4) -> Scope38/1
  Tinitial5/1 -> Integrator7/2
  Bedroom1/5(Out5) -> [Mdot_Actual_6]
  Bedroom1/1(Out1) -> [T_return_R6]
  [MassFlow_Full_Open_6] -> Bedroom1/18(In18)
  Twall110/1 -> Subsystem30/3(In3)
  Subsystem8/3(Out3) -> Bedroom1/10(In10)
  Subsystem8/2(Out2) -> Bedroom1/9(In9)
  Subsystem8/5(Out5) -> Bedroom1/12(In12)
  Twall35/1 -> Subsystem8/5(In5)
  Twall32/1 -> Subsystem8/2(In2)
  Twall111/1 -> Subsystem30/4(In4)
  Twall74/1 -> Subsystem19/1(In1)
  Diffuse Irradiance5/1 -> Bedroom1/17(In17)
  Twall33/1 -> Subsystem8/3(In3)
  Subsystem8/4(Out4) -> Bedroom1/11(In11)
  Subsystem30/1(Out1) -> Bedroom1/6(In6)
  Bedroom1/2(Out2) -> Terminator4/1
  Twall109/1 -> Subsystem30/2(In2)
  Subsystem30/2(Out2) -> Bedroom1/7(In7)

== system Final_Model_Building_2_AirflowAdded_BufferMode/Subsystem_Room7 ==
  Bedroom 2 : Subsystem
      mask Display:
      | port_label('input', 1, 'THB in')
      | port_label('input', 2, 'T In')
      | port_label('input', 3, 'T Out')
      | port_label('input', 4, 'T up (conv)')
      | port_label('input', 5, 'T Down (conv)')
      | port_label('input', 6, 'T Bel (cond)')
      | port_label('input', 7, 'T Abv (cond)')
      | port_label('input', 8, 'T N1')
      | port_label('input', 9, 'T N2')
      | port_label('input', 10, 'T N3')
      | port_label('input', 11, 'T N4')
      | port_label('input', 12, 'T N5')
      | port_label('input', 13, 'T Wall')
      | port_label('input', 14, 'Ang')
      | port_label('input', 15, 'Tilt')
      | port_label('input', 16, 'DNI')
      | port_label('input', 17, 'DiffI')
      | 
      | port_label('output', 1, 'THB Out')
      | port_label('output', 2, 'DeltaT Wall')
      | port_label('output', 3, 'DeltaT Room')
      | 
      | port_label('input', 18, 'm_dot_Fully_open')
      | port_label('output', 5, 'm_dot_Actual')
  DNI6 : Constant  Value=0
  Diffuse Irradiance6 : Constant  Value=0
  Ground9 : Ground
  Incidence Angle6 : Constant  Value=60
  Integrator11 : Integrator  InitialConditionSource=external  InitialCondition=Tin1
  Panel TIlt6 : Constant  Value=90
  Scope37 : Scope
  Subsystem20 : Subsystem
      mask Display:
      | disp('Vertical \n Convective \n Signalling \n Block')
      | port_label('input', 1, 'Nbr1')
      | port_label('input', 2, 'Nbr2')
      | 
      | port_label('output', 1, 'Tup')
      | port_label('output', 2, 'Tdwn')
  Subsystem25 : Subsystem
      mask Display:
      | disp('Vertical \n Conductive \n Signalling \n Block')
      | port_label('input', 1, 'Bel1')
      | port_label('input', 2, 'Bel2')
      | port_label('input', 3, 'Abv1')
      | port_label('input', 4, 'Abv2')
      | 
      | port_label('output', 1, 'T Bel')
      | port_label('output', 2, 'T Abv')
  Subsystem9 : Subsystem
      mask Display:
      | disp('Horizontal \n Neighbour \n Signalling \n Block')
      | port_label('input', 1, 'Nbr1')
      | port_label('input', 2, 'Nbr2')
      | port_label('input', 3, 'Nbr3')
      | port_label('input', 4, 'Nbr4')
      | port_label('input', 5, 'Nbr5')
      | port_label('output', 1, 'TN1')
      | port_label('output', 2, 'TN2')
      | port_label('output', 3, 'TN3')
      | port_label('output', 4, 'TN4')
      | port_label('output', 5, 'TN5')
  Terminator3 : Terminator
  Tinitial6 : Constant  Value=20
  Twall36 : Constant  Value=neighbourMatrix(1,7)
  Twall37 : Constant  Value=neighbourMatrix(2,7)
  Twall38 : Constant  Value=neighbourMatrix(3,7)
  Twall39 : Constant  Value=neighbourMatrix(4,7)
  Twall40 : Constant  Value=neighbourMatrix(5,7)
  Twall76 : Constant  Value=convUDMatrix(1,7)
  Twall77 : Constant  Value=convUDMatrix(2,7)
  Twall88 : Constant  Value=condUDMatrix(1,7)
  Twall89 : Constant  Value=condUDMatrix(2,7)
  Twall90 : Constant  Value=condUDMatrix(3,7)
  Twall91 : Constant  Value=condUDMatrix(4,7)
  tag scope: DeltaT_7=global, Mdot_Actual_7=global, T_7=global, T_return_R7=global
  wires:
  Panel TIlt6/1 -> Bedroom 2/15(In15)
  [T_Out] -> Bedroom 2/3(In3)
  Twall36/1 -> Subsystem9/1(In1)
  Bedroom 2/3(Out3) -> [DeltaT_7]
  [MassFlow_Full_Open_7] -> Bedroom 2/18(In18)
  Diffuse Irradiance6/1 -> Bedroom 2/17(In17)
  Bedroom 2/1(Out1) -> [T_return_R7]
  Bedroom 2/2(Out2) -> Terminator3/1
  Twall88/1 -> Subsystem25/1(In1)
  Subsystem9/3(Out3) -> Bedroom 2/10(In10)
  Bedroom 2/5(Out5) -> [Mdot_Actual_7]
  Twall90/1 -> Subsystem25/3(In3)
  Subsystem25/2(Out2) -> Bedroom 2/7(In7)
  Incidence Angle6/1 -> Bedroom 2/14(In14)
  DNI6/1 -> Bedroom 2/16(In16)
  Integrator11/1 -> [T_7]
  Subsystem9/1(Out1) -> Bedroom 2/8(In8)
  Subsystem25/1(Out1) -> Bedroom 2/6(In6)
  [DeltaT_7] -> Integrator11/1
  Twall40/1 -> Subsystem9/5(In5)
  Subsystem20/1(Out1) -> Bedroom 2/4(In4)
  Tinitial6/1 -> Integrator11/2
  Twall37/1 -> Subsystem9/2(In2)
  Subsystem20/2(Out2) -> Bedroom 2/5(In5)
  Bedroom 2/4(Out4) -> Scope37/1
  [THB_In] -> Bedroom 2/1(In1)
  Twall76/1 -> Subsystem20/1(In1)
  Subsystem9/4(Out4) -> Bedroom 2/11(In11)
  [T_7] -> Bedroom 2/2(In2)
  Subsystem9/2(Out2) -> Bedroom 2/9(In9)
  Twall39/1 -> Subsystem9/4(In4)
  Twall89/1 -> Subsystem25/2(In2)
  Ground9/1 -> Bedroom 2/13(In13)
  Twall38/1 -> Subsystem9/3(In3)
  Subsystem9/5(Out5) -> Bedroom 2/12(In12)
  Twall91/1 -> Subsystem25/4(In4)
  Twall77/1 -> Subsystem20/2(In2)
